simulink model "relay"  (R2021b)
settings: Solver=VariableStepAuto  StartTime=0.0  StopTime=3  RelTol=1e-3
undefined symbols (not defined in the file): Angeln, DiscIntNeverNeededParam, J, ke, km, L, Moth, R, U
settings Model: Creator=vital  LastModifiedBy=vital
settings SolverCC: AlgebraicLoopSolver=TrustRegion
settings DebuggingCC: SFMachineParentedDataDiag=warning

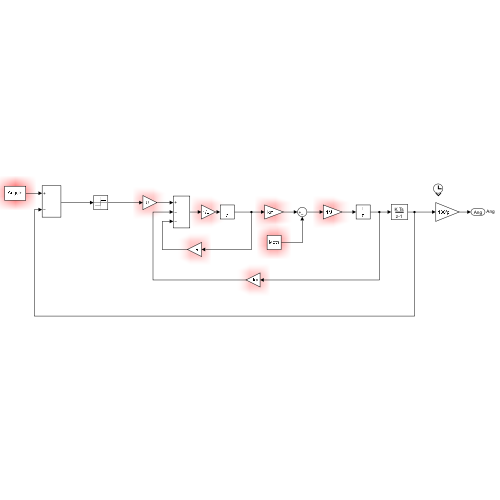
[thumbnail: Simulink's stored preview of the top-level diagram]
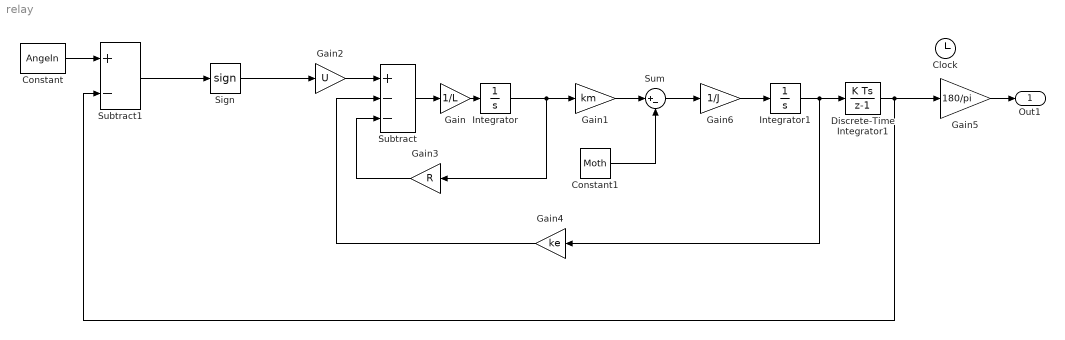
== system relay ==
  Clock : Clock
  Constant : Constant  Value=Angeln
  Constant1 : Constant  Value=Moth
  Discrete-Time Integrator1 : DiscreteIntegrator  SampleTime=0.01  ICPrevOutput=DiscIntNeverNeededParam  ICPrevScaledInput=DiscIntNeverNeededParam
  Gain : Gain  Gain=1/L
  Gain1 : Gain  Gain=km
  Gain2 : Gain  Gain=U
  Gain3 : Gain  Gain=R
  Gain4 : Gain  Gain=ke
  Gain5 : Gain  Gain=180/pi
  Gain6 : Gain  Gain=1/J
  Integrator : Integrator
  Integrator1 : Integrator
  Sign : Signum
  Subtract : Sum  Inputs=+--
  Subtract1 : Sum  Inputs=+-
  Sum : Sum  Inputs=|+-
  Out1 : Outport  SignalName=Ang
  wires:
  Subtract/1 -> Gain/1
  Gain/1 -> Integrator/1
  Integrator/1 -> Gain3/1, Gain1/1
  Gain3/1 -> Subtract/3
  Integrator1/1 -> Gain4/1, Discrete-Time Integrator1/1
  Gain4/1 -> Subtract/2
  Subtract1/1 -> Sign/1
  Gain2/1 -> Subtract/1
  Constant/1 -> Subtract1/1
  Gain5/1 -> Out1/1
  Discrete-Time Integrator1/1 -> Subtract1/2, Gain5/1
  Sign/1 -> Gain2/1
  Gain1/1 -> Sum/1
  Sum/1 -> Gain6/1
  Constant1/1 -> Sum/2
  Gain6/1 -> Integrator1/1
